simulink model "sine_Wave_question1"  (R2023b)
settings: Solver=FixedStepAuto  StartTime=0.0  StopTime=10.0  RelTol=1e-3
settings Model: Creator=Pranav  LastModifiedBy=Pranav

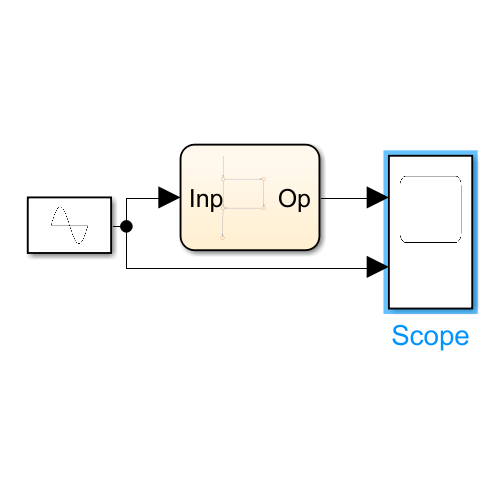
[thumbnail: Simulink's stored preview of the top-level diagram]
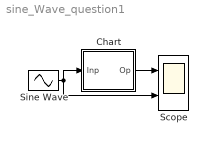
== system sine_Wave_question1 ==
  Chart : Stateflow chart  TreatAsAtomicUnit=on
  Scope : Scope  NumInputPorts=2
  Sine Wave : Sin  SampleTime=0
  wires:
  Sine Wave/1 -> Scope/2, Chart/1(Inp)
  Chart/1(Op) -> Scope/1

== stateflow chart sine_Wave_question1/Chart ==
  (default) -> (junction 1)
  (junction 1) -> (junction 3) [order 1] : [Inp>=0]
  (junction 1) -> (junction 8) [order 2] : {Op=-1;}
  (junction 3) -> (junction 5) : {Op=1;}
  (junction 5) -> (junction 8)
  (junction 8) -> (junction 16)
  data: Inp input; Op output
